simulink model "Lab3"  (R2023b)
settings: Solver=ode5  StartTime=0  StopTime=800  FixedStep=0.01  RelTol=1e-3
values from neighbouring files (symbols this model uses):
  I = diag(Iv)    [InitDoubleSpin.m]    (also in InitLab03.m)
  invI = inv(I)    [InitDoubleSpin.m]    (also in InitLab03.m)
  w0 = [1e-6; 0.005; 0.2]    [InitDoubleSpin.m]    (also in InitLab03.m = [2*pi; 0.5; 1])
libraries: matrix_library x1
settings Model: Creator=elisa  LastModifiedBy=elisa

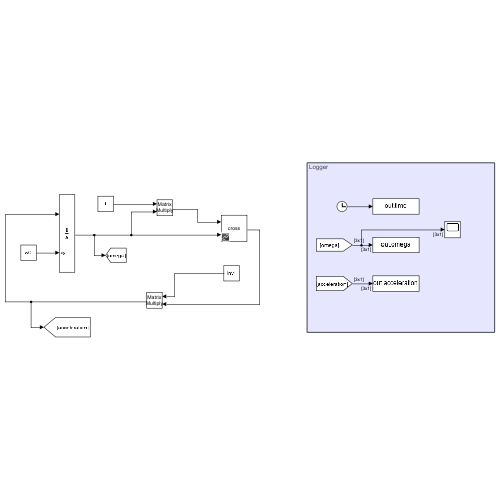
[thumbnail: Simulink's stored preview of the top-level diagram]
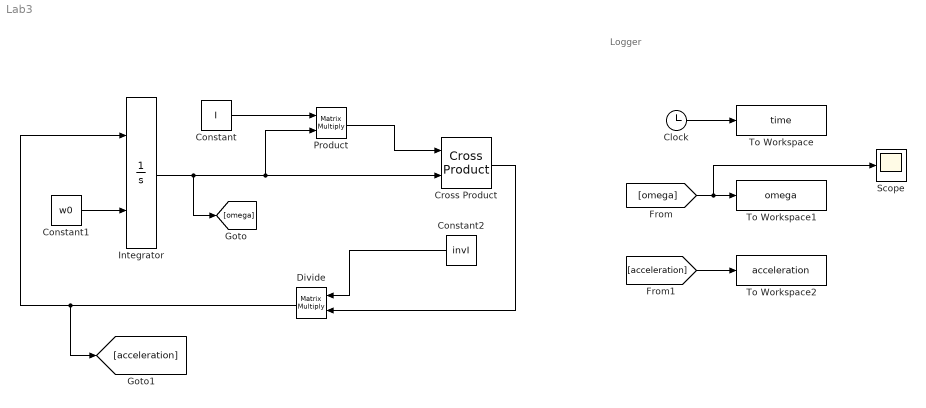
== system Lab3 ==
  note: Logger
  Clock : Clock
  Constant : Constant  Value=I
  Constant1 : Constant  Value=w0  VectorParams1D=off
  Constant2 : Constant  Value=invI
  Cross Product : matrix_library/Cross Product
  Divide : Product  Inputs=**  Multiplication=Matrix(*)
  Integrator : Integrator  InitialConditionSource=external
  Product : Product  Multiplication=Matrix(*)
  Scope : Scope
  To Workspace : ToWorkspace  VariableName=time  SaveFormat=Timeseries  SampleTime=-1
  To Workspace1 : ToWorkspace  VariableName=omega  SaveFormat=Timeseries  SampleTime=-1
  To Workspace2 : ToWorkspace  VariableName=acceleration  SaveFormat=Timeseries  SampleTime=-1
  wires:
  Constant1/1 -> Integrator/2
  Constant/1 -> Product/1
  Integrator/1 -> [omega], Product/2, Cross Product/2
  Product/1 -> Cross Product/1
  Divide/1 -> [acceleration], Integrator/1
  Clock/1 -> To Workspace/1
  [omega] -> Scope/1, To Workspace1/1
  [acceleration] -> To Workspace2/1
  Constant2/1 -> Divide/1
  Cross Product/1 -> Divide/2
